simulink model "pca10040_demo"  (Simulink 7.3)
settings: Solver=ode3  SolverMode=SingleTasking  StartTime=0.0  StopTime=10.0  RelTol=1e-3
PreLoadFcn:
  | waijung.modelPreload; % Required for working with Waijung Blockset. Do not remove.
undefined symbols (not defined in the file): Blocking, In1, In2, Non, nRF52832QFAA, Out1, Out2, S132, v6
libraries: nrf5_ble_lib x4, waijung_string_manipulate x4, simulink x3, nrf5_io_lib x2, nrf5_device_config_lib x1
CloseFcn:
  | waijung.modelClose; % Required for working with Waijung Blockset. Do not remove.
settings Model: Creator=Krisada  LastModifiedBy=Navy
settings OptimizationCC: OptimizeModelRefInitCode=on  LifeSpan=1
settings HardwareCC: ProdEndianess=LittleEndian  ProdHWDeviceType=ARM Compatible->Cortex - M0  TargetEndianess=LittleEndian  TargetHWDeviceType=ARM Compatible->Cortex - M0
settings RTWCC: SystemTargetFile=nrf5.tlc  GenerateMakefile=off  TemplateMakefile=ert_default_tmf  Description=nRF5 Target  ProcessScript=nrf5_make_rtw_hook
settings CodeAppCC: IgnoreCustomStorageClasses=off
settings STFCustomTargetCC: ModelReferenceCompliant=off  CombineOutputUpdateFcns=on  ERTCustomFileBanners=on  SupportContinuousTime=off  SupportNonInlinedSFcns=off  SystemTargetFile=nrf5.tlc
settings ERTTargetCC: MultiwordLength=2048  ModelReferenceCompliant=off  ParMdlRefBuildCompliant=off  CompOptLevelCompliant=off  ERTFirstTimeCompliant=off  ModelStepFunctionPrototypeControlCompliant=off  CPPClassGenCompliant=off  InlinedParameterPlacement=NonHierarchical  ERTSrcFileBannerTemplate=nrf5_code_template.cgt  ERTHdrFileBannerTemplate=nrf5_code_template.cgt  ERTDataSrcFileTemplate=nrf5_code_template.cgt  ERTDataHdrFileTemplate=nrf5_code_template.cgt  ERTCustomFileTemplate=nrf5_file_process.tlc

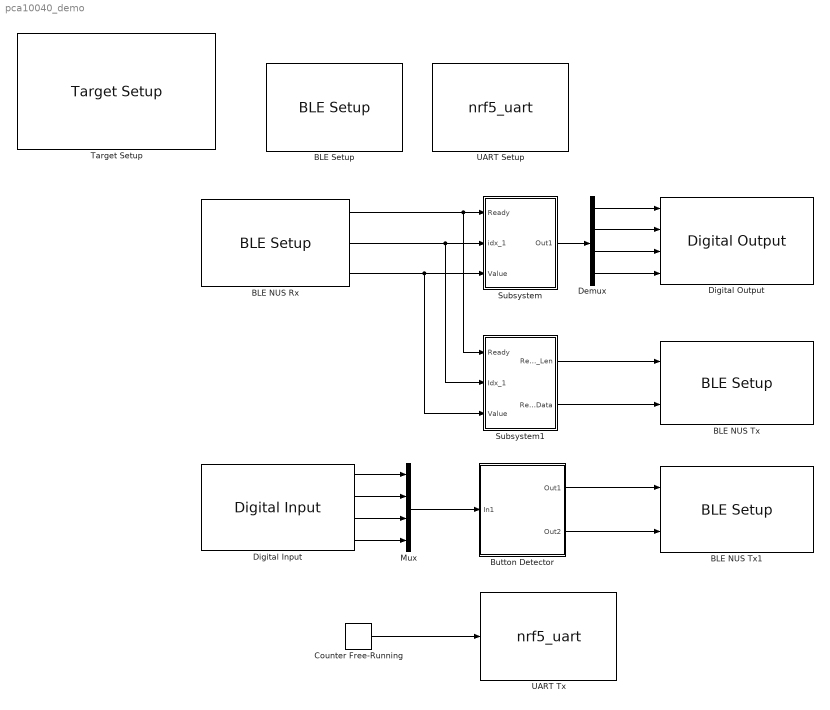
== system pca10040_demo ==
  BLE NUS Rx : nrf5_ble_lib/BLE Setup  conf=Rx  bleprofile=NUS  ble_secure_dfu=off  ble_secure_dfu_public_key='123bd49bffb387f1de3dc8dc1fc8fcce952739d331fafeb7dd16837154ace7994a0a05af319f68e2a07478477b8db746643d6dd7f5f191193738984ffcd2b963'  devicename='Nordic_UART'  advanceoptions=on  rxbuffersize=64  txbuffersize=64  transfer=Non-Blocking  packetmode=Ascii  binheader='7E 7E'  binterminator='03 03'  porttype_double=0  porttype_single=0  porttype_int8=0  porttype_uint8=3  porttype_int16=0  porttype_uint16=0  porttype_int32=0  porttype_uint32=2  asciiformat='led%d=%d'  rx_asciiterminator="CRLF (0x0D 0x0A - \"\\r\\n\")"  tx_asciiterminator=None  storagename=<empty>  portpinstr=0  sampletime=-1  enablecustomportlabel=off  cinputportlabel=In1,In2  coutputportlabel=Out1,Out2  blockid=BLENUSRx  inputporttype=[]  inputportwidth=[]  inputportlabel={}  outputporttype=[3 6 6]  outputportwidth=[]  outputportlabel={'READY' 'int32' 'int32'}  compat=0  optionstring1="[\"64\",\"64\",\"Non-Blocking\",\"Ascii\",\"led%d=%d\",\"0x0D, 0x0A\",\"2\",\"NUS\",\"Nordic_UART\",\"1\",\"0\"]"  optionstring2="[\"int32_t\",\"int32_t\"]"  optionstring3="[\"0x7E\",\"0x7E\"]"  optionstring4="[\"0x3\",\"0x3\"]"
  BLE NUS Tx : nrf5_ble_lib/BLE Setup  conf=Tx  bleprofile=NUS  ble_secure_dfu=off  ble_secure_dfu_public_key='123bd49bffb387f1de3dc8dc1fc8fcce952739d331fafeb7dd16837154ace7994a0a05af319f68e2a07478477b8db746643d6dd7f5f191193738984ffcd2b963'  devicename='Nordic_UART'  advanceoptions=on  rxbuffersize=64  txbuffersize=64  transfer=Blocking  packetmode=Raw Buffer  binheader='7E 7E'  binterminator='03 03'  porttype_double=0  porttype_single=0  porttype_int8=0  porttype_uint8=3  porttype_int16=0  porttype_uint16=0  porttype_int32=0  porttype_uint32=2  asciiformat='led%d=%d'  rx_asciiterminator="CRLF (0x0D 0x0A - \"\\r\\n\")"  tx_asciiterminator=None  storagename=<empty>  portpinstr=0  sampletime=-1  enablecustomportlabel=off  cinputportlabel=In1,In2  coutputportlabel=Out1,Out2  blockid=BLENUSTx  inputporttype=[5 3]  inputportwidth=[1 -1]  inputportlabel={'Len','Data'}  outputporttype=[]  outputportwidth=[]  outputportlabel={}  compat=0  optionstring1="[\"64\",\"64\",\"Blocking\",\"Raw Buffer\",\"led%d=%d\",\"\",\"\",\"NUS\",\"Nordic_UART\",\"1\",\"0\"]"  optionstring2="[\"int32_t\",\"int32_t\"]"  optionstring3="[\"0x7E\",\"0x7E\"]"  optionstring4="[\"0x3\",\"0x3\"]"
  BLE NUS Tx1 : nrf5_ble_lib/BLE Setup  conf=Tx  bleprofile=NUS  ble_secure_dfu=off  ble_secure_dfu_public_key='123bd49bffb387f1de3dc8dc1fc8fcce952739d331fafeb7dd16837154ace7994a0a05af319f68e2a07478477b8db746643d6dd7f5f191193738984ffcd2b963'  devicename='Nordic_UART'  advanceoptions=on  rxbuffersize=64  txbuffersize=64  transfer=Blocking  packetmode=Raw Buffer  binheader='7E 7E'  binterminator='03 03'  porttype_double=0  porttype_single=0  porttype_int8=0  porttype_uint8=3  porttype_int16=0  porttype_uint16=0  porttype_int32=0  porttype_uint32=2  asciiformat='Btn:%u,%u,%u,%u'  rx_asciiterminator="CRLF (0x0D 0x0A - \"\\r\\n\")"  tx_asciiterminator=None  storagename=<empty>  portpinstr=0  sampletime=-1  enablecustomportlabel=off  cinputportlabel=In1,In2  coutputportlabel=Out1,Out2  blockid=BLENUSTx1  inputporttype=[5 3]  inputportwidth=[1 -1]  inputportlabel={'Len','Data'}  outputporttype=[]  outputportwidth=[]  outputportlabel={}  compat=0  optionstring1="[\"64\",\"64\",\"Blocking\",\"Raw Buffer\",\"Btn:%u,%u,%u,%u\",\"\",\"\",\"NUS\",\"Nordic_UART\",\"1\",\"0\"]"  optionstring2="[\"uint32_t\",\"uint32_t\",\"uint32_t\",\"uint32_t\"]"  optionstring3="[\"0x7E\",\"0x7E\"]"  optionstring4="[\"0x3\",\"0x3\"]"
  BLE Setup : nrf5_ble_lib/BLE Setup  conf=Setup  bleprofile=NUS  ble_secure_dfu=off  ble_secure_dfu_public_key='123bd49bffb387f1de3dc8dc1fc8fcce952739d331fafeb7dd16837154ace7994a0a05af319f68e2a07478477b8db746643d6dd7f5f191193738984ffcd2b963'  devicename='aMG_BLE Demo'  advanceoptions=on  rxbuffersize=64  txbuffersize=64  transfer=Blocking  packetmode=Ascii  binheader='7E 7E'  binterminator='03 03'  porttype_double=0  porttype_single=0  porttype_int8=0  porttype_uint8=3  porttype_int16=0  porttype_uint16=0  porttype_int32=0  porttype_uint32=2  asciiformat='Value=%1.2f'  rx_asciiterminator="CRLF (0x0D 0x0A - \"\\r\\n\")"  tx_asciiterminator=None  storagename=<empty>  portpinstr=0  sampletime=-1  enablecustomportlabel=off  cinputportlabel=In1,In2  coutputportlabel=Out1,Out2  blockid=BLESetup  inputporttype=[]  inputportwidth=[]  inputportlabel={}  outputporttype=[]  outputportwidth=[]  outputportlabel={}  compat=0  optionstring1="[\"64\",\"64\",\"Blocking\",\"Ascii\",\"Value=%1.2f\",\"\",\"\",\"NUS\",\"aMG_BLE Demo\",\"1\",\"0\"]"  optionstring2="[\"float\"]"  optionstring3="[\"0x7E\",\"0x7E\"]"  optionstring4="[\"0x3\",\"0x3\"]"
  Button Detector : Subsystem
  Counter Free-Running : simulink/Sources/Counter Free-Running  SystemSampleTime=-1  NumBits=32  tsamp=-1
  Demux : Demux
  Digital Input : nrf5_io_lib/Digital Input  conf=input  port=0  drivemode=High  outputpintype=Open Drain  inputpintype=Pull Up  usepin0=off  usepin1=off  usepin2=off  usepin3=off  usepin4=off  usepin5=off  usepin6=off  usepin7=off  usepin8=off  usepin9=off  usepin10=off  usepin11=off  usepin12=off  usepin13=on  usepin14=on  usepin15=on  usepin16=on  usepin17=off  usepin18=off  usepin19=off  usepin20=off  usepin21=off  usepin22=off  usepin23=off  usepin24=off  usepin25=off  usepin26=off  usepin27=off  usepin28=off  usepin29=off  usepin30=off  usepin31=off  outputmode=uint8  sampletime=-1  enablecustomportlabel=off  cinputportlabel=In1,In2  coutputportlabel=Out1,Out2  portpinstr=off  blockid=DigitalInput  inputporttype=[]  inputportwidth=[]  inputportlabel={}  outputporttype=[3,3,3,3]  outputportwidth=[]  outputportlabel={'P0.13','P0.14','P0.15','P0.16'}  compat=0  optionstring="[\"0\",\"High\",\"PULLUP\",\"H0D1\",\"dummy\",\"dummy\",\"dummy\",\"dummy\",\"dummy\",\"dummy\",\"off\",\"off\",\"off\",\"off\",\"off\",\"off\",\"off\",\"off\",\"off\",\"off\",\"off\",\"off\",\"off\",\"on\",\"on\",\"on\",\"on\",\"off\",\"off\",\"off\",\"off\",\"off\",\"off\",\"off\",\"off\",\"off\",\"off\",\"off\",\"off\",\"off\",\"off\",\"off\"]"
  Digital Output : nrf5_io_lib/Digital Output  conf=output  port=0  drivemode=High  outputpintype=Push Pull  inputpintype=None  usepin0=off  usepin1=off  usepin2=off  usepin3=off  usepin4=off  usepin5=off  usepin6=off  usepin7=off  usepin8=off  usepin9=off  usepin10=off  usepin11=off  usepin12=off  usepin13=off  usepin14=off  usepin15=off  usepin16=off  usepin17=on  usepin18=on  usepin19=on  usepin20=on  usepin21=off  usepin22=off  usepin23=off  usepin24=off  usepin25=off  usepin26=off  usepin27=off  usepin28=off  usepin29=off  usepin30=off  usepin31=off  outputmode=uint8  sampletime=-1  enablecustomportlabel=off  cinputportlabel=In1,In2  coutputportlabel=Out1,Out2  portpinstr=off  blockid=DigitalOutput  inputporttype=[-1,-1,-1,-1]  inputportwidth=[]  inputportlabel={'P0.17','P0.18','P0.19','P0.20'}  outputporttype=[]  outputportwidth=[]  outputportlabel={}  compat=0  optionstring="[\"0\",\"High\",\"NOPULL\",\"H0H1\",\"dummy\",\"dummy\",\"dummy\",\"dummy\",\"dummy\",\"dummy\",\"off\",\"off\",\"off\",\"off\",\"off\",\"off\",\"off\",\"off\",\"off\",\"off\",\"off\",\"off\",\"off\",\"off\",\"off\",\"off\",\"off\",\"on\",\"on\",\"on\",\"on\",\"off\",\"off\",\"off\",\"off\",\"off\",\"off\",\"off\",\"off\",\"off\",\"off\",\"off\"]"
  Mux : Mux
  Subsystem : Subsystem
  Subsystem1 : Subsystem
  Target Setup : nrf5_device_config_lib/Target Setup  Priority=100  compiler=GNU ARM  previous_compiler=GNU ARM  mcu=nRF52832QFAA (S132-v6)  family=nrf52  softdevice=S132  clockconfig=None  system_nrf5_c_path=c:\users\Krisada\desktop\waijung\waijung-subversion-trunk\targets\nrf5_target\nrf5\utils\nrf5_lib\inc  lowpower=on  showmemoryconfiguration=on  stacksize=0x1000  heapsize=0x00  enableautocompiledownload=on  fullchiperase=off  ble_secure_dfu=off  ble_secure_dfu_public_key='123bd49bffb387f1de3dc8dc1fc8fcce952739d331fafeb7dd16837154ace7994a0a05af319f68e2a07478477b8db746643d6dd7f5f191193738984ffcd2b963'  programmerinterface=nrfjprog  editctrlstr=on  compilercontrolstr=-O3 -g3 -mcpu=cortex-m4 -mthumb -mabi=aapcs -Wall -mfloat-abi=hard -mfpu=fpv4-sp-d16 -ffunction-sections -fdata-sections -fno-strict-aliasing -fno-builtin -fshort-enums  assemblercontrolstr=-O3 -g3 -mcpu=cortex-m4 -mthumb -mabi=aapcs -mfloat-abi=hard -mfpu=fpv4-sp-d16  linkercontrolstr=-O3 -g3 -mthumb -mabi=aapcs -mcpu=cortex-m4 -mfloat-abi=hard -mfpu=fpv4-sp-d16 -Wl,--gc-sections --specs=nano.specs  global_define=CONFIG_GPIO_AS_PINRESET,FLOAT_ABI_HARD,NRF52,NRF52832_XXAA,NRF52_PAN_74,S132,SOFTDEVICE_PRESENT,SWI_DISABLE0,NRF_SD_BLE_API_VERSION=6  runafterdownload=on  execprofile=None  profileruart=3  profilerbaud=500000  profilertxpin=D8  profilerinitstr=0.01,168000000,1680000,500000,0  manualsetsampletime=on  sampletime=0.1  blockid=TargetSetup  systickreloadvalue=10  hseval=8000000  lastprofileruart=3  hclk=168000000  flashorigin=0x26000  flashlength=256k  ramorigin=0x200032C8  ramlength=51k  useextram=off  optionstring="[\"s132\",\"on\"]"
  UART Setup : S-Function  FunctionName=nrf5_uart  Parameters=conf,inputporttype,inputportwidth,outputporttype,outputportwidth,optionstring1,optionstring2,optionstring3,optionstring4,sampletime,blockid  EnableBusSupport=off  mask(nrf5_uart){conf=Setup, uartmodule=0, baudrate=115200, databits=8, parity=None, stopbit=1, txpin=P0.6, rxpin=P0.8, flowcontrol=None, ctspin=P0.4, rtspin=P0.2, advanceoptions=on, rxbuffersize=64, txbuffersize=64, transfer=Blocking, packetmode=Binary, binheader='7E 7E', binterminator='03 03', porttype_double=0, porttype_single=0, porttype_int8=0, porttype_uint8=0, porttype_int16=0, porttype_uint16=0, porttype_int32=0, porttype_uint32=2, asciiformat='Value=%1.2f', rx_asciiterminator=CR (0x0D - "\r"), tx_asciiterminator=CR (0x0D - "\r"), storagename=<empty>, portpinstr=0, sampletime=-1, enablecustomportlabel=off, cinputportlabel=In1,In2, coutputportlabel=Out1,Out2, blockid=UARTSetup, inputporttype=[], inputportwidth=[], inputportlabel={}, outputporttype=[], outputportwidth=[], outputportlabel={}, compat=0, optionstring1=["0","115200","6","8","None","4","2","64","64","Blocking","Binary","","0","","0","Value=%1.2f","","",""], optionstring2=["float"], optionstring3=["0x7E","0x7E"], optionstring4=["0x3","0x3"]}
      mask prompts: conf "Configuration"; uartmodule "UART Module"; baudrate "Baud rate (bps)"; databits "Data bits"; stopbit "Stop bit"; txpin "Tx Pin"; rxpin "Rx Pin"; flowcontrol "Hardware flow control"; ctspin "HW Flow control, CTS Pin"; rtspin "HW Flow control, RTS Pin"; advanceoptions "Advance options"; rxbuffersize "Rx buffer size (bytes)"; txbuffersize "Tx buffer size (bytes)"; packetmode "Packet mode"; binheader "Binary header (example: '7E 7E')"; binterminator "Binary terminator (example: '03 03')"; porttype_double "Number of data port, type DOUBLE"; porttype_single "Number of data port, type SINGLE"; porttype_int8 "Number of data port, type INT8"; porttype_uint8 "Number of data port, type UINT8"; porttype_int16 "Number of data port, type INT16"; porttype_uint16 "Number of data port, type UINT16"; porttype_int32 "Number of data port, type INT32"; porttype_uint32 "Number of data port, type UINT32"; asciiformat "Ascii format"; rx_asciiterminator "End of packet"; tx_asciiterminator "End of packet"; storagename "Buffer"; portpinstr "Port Pin String"; sampletime "Sample time (sec)"; enablecustomportlabel "Enable custom port labels"; cinputportlabel "Custom input port labels (Ex. In1, In2, In3)"; coutputportlabel "Custom output port labels (Ex. Out1, Out2, Out3)"; blockid "Block ID"; inputporttype "Input Port Type"; inputportwidth "Input Port Width"; inputportlabel "Input Port Label"; outputporttype "Output Port Type"; outputportwidth "Output Port Width"; outputportlabel "Output port label"; compat "Compatibility (Reserved for future use)"; optionstring1 "String(s) to be passed to TLC"; optionstring2 "String(s) to be passed to TLC"; optionstring3 "String(s) to be passed to TLC"; optionstring4 "String(s) to be passed to TLC"
      mask help:
      | UART Setup block.
      | Baud rate:
      |  - Valid value is 1200 to 1000000.
      mask init:
      | nrf5_uart_callback('init');
      mask Help: web(fullfile(waijungdocroot,'nrf5_uart_setup.htm'), '-browser')
      mask StyleString: popup(Setup|Tx|Rx),popup(0),edit,popup(8),popup(None|Odd|Even),popup(0.5|1|1.5|2),popup(Not used|P0.0|P0.1|P0.2|P0.3|P0.4|P0.5|P0.6|P0.7|P0.8|P0.9|P0.10|P0.11|P0.12|P0.13|P0.14|P0.15|P0.16|P0.17|P0.18|P0.19|P0.20|P0.21|P0.22|P0.23|P0.24|P0.25|P0.26|P0.27|P0.28|P0.29|P0.30|P0.31),popup(Not used|P0.0|P0.1|P0.2|P0.3|P0.4|P0.5|P0.6|P0.7|P0.8|P0.9|P0.10|P0.11|P0.12|P0.13|P0.14|P0.15|P0.16|P0.17|P0.18|P0.19|P0.20|P0.21|P0.22|P0.23|P0.24|P0.25|P0.26|P0.27|P0.28|P0.29|P0.30|P0.31),popup(None|RTS/CTS),popup(P0.0|P0.1|P0.2|P0.3|P0.4|P0.5|P0.6|P0.7|P0.8|P0.9|P0.10|P0.11|P0.12|P0.13|P0.14|P0.15|P0.16|P0.17|P0.18|P0.19|P0.20|P0.21|P0.22|P0.23|P0.24|P0.25|P0.26|P0.27|P0.28|P0.29|P0.30|P0.31),popup(P0.0|P0.1|P0.2|P0.3|P0.4|P0.5|P0.6|P0.7|P0.8|P0.9|P0.10|P0.11|P0.12|P0.13|P0.14|P0.15|P0.16|P0.17|P0.18|P0.19|P0.20|P0.21|P0.22|P0.23|P0.24|P0.25|P0.26|P0.27|P0.28|P0.29|P0.30|P0.31),checkbox,popup(16|32|64|128|256|512|1024),popup(16|32|64|128|256|512|1024),popup(Blocking|Non-Blocking),popup(Ascii|Binary|String Buffer),edit,edit,edit,edit,edit,edit,edit,edit,edit,edit,edit,popup(CR (0x0D - "\r")|LF (0x0A - "\n")|CRLF (0x0D 0x0A - "\r\n")),popup(CR (0x0D - "\r")|LF (0x0A - "\n")|CRLF (0x0D 0x0A - "\r\n")|None),popup(<empty>),edit,edit,checkbox,edit,edit,edit,edit,edit,edit,edit,edit,edit,edit,edit,edit,edit,edit
      mask CallbackString: nrf5_uart_callback('conf');||||||||nrf5_uart_callback('flowcontrol');|||nrf5_uart_callback('advanceoptions');|||nrf5_uart_callback('transfer');|nrf5_uart_callback('packetmode');|nrf5_uart_callback('binheader');|nrf5_uart_callback('binterminator');|nrf5_uart_callback('updateport');|nrf5_uart_callback('updateport');|nrf5_uart_callback('updateport');|nrf5_uart_callback('updateport');|nrf5_uart_callback('updateport');|nrf5_uart_callback('updateport');|nrf5_uart_callback('updateport');|nrf5_uart_callback('updateport');|nrf5_uart_callback('asciiformat');|||||nrf5_uart_callback('sampletime');|nrf5_uart_callback('enablecustomportlabel');|||nrf5_uart_callback('blockid');|||||||||||
      mask Display: text(0.5, 0.5, '[UART0_Setup]\nBaud: 115200\nTx/Rx buffer: 64/64\nTx/Rx pin: P0.6/P0.8','ver','middle','hor','center');
  UART Tx : S-Function  FunctionName=nrf5_uart  Parameters=conf,inputporttype,inputportwidth,outputporttype,outputportwidth,optionstring1,optionstring2,optionstring3,optionstring4,sampletime,blockid  EnableBusSupport=off  mask(nrf5_uart){conf=Tx, uartmodule=0, baudrate=115200, databits=8, parity=None, stopbit=1, txpin=P0.2, rxpin=P0.3, flowcontrol=None, ctspin=P0.4, rtspin=P0.2, advanceoptions=on, rxbuffersize=64, txbuffersize=64, transfer=Blocking, packetmode=Ascii, buffersize=32, binheader='7E 7E', binterminator='03 03', porttype_double=0, porttype_single=0, porttype_int8=0, porttype_uint8=0, porttype_int16=0, porttype_uint16=0, porttype_int32=0, porttype_uint32=2, asciiformat='Running=%u', rx_asciiterminator=CR (0x0D - "\r"), tx_asciiterminator=CRLF (0x0D 0x0A - "\r\n"), storagename=<empty>, portpinstr=0, sampletime=0.1, enablecustomportlabel=off, cinputportlabel=In1,In2, coutputportlabel=Out1,Out2, blockid=UARTTx, inputporttype=[-1], inputportwidth=[], inputportlabel={'uint32'}, outputporttype=[], outputportwidth=[], outputportlabel={}, compat=0, optionstring1=["0","115200","2","3","None","4","2","64","64","Blocking","Ascii","","0","","0","Running=%u","0x0D, 0x0A","2",""], optionstring2=["uint32_t"], optionstring3=["0x7E","0x7E"], optionstring4=["0x3","0x3"]}
      mask prompts: conf "Configuration"; uartmodule "UART Module"; baudrate "Baud rate (bps)"; databits "Data bits"; stopbit "Stop bit"; txpin "Tx Pin"; rxpin "Rx Pin"; flowcontrol "Hardware flow control"; ctspin "HW Flow control, CTS Pin"; rtspin "HW Flow control, RTS Pin"; advanceoptions "Advance options"; rxbuffersize "Rx buffer size (bytes)"; txbuffersize "Tx buffer size (bytes)"; packetmode "Packet mode"; buffersize "Buffer size"; binheader "Binary header (example: '7E 7E')"; binterminator "Binary terminator (example: '03 03')"; porttype_double "Number of data port, type DOUBLE"; porttype_single "Number of data port, type SINGLE"; porttype_int8 "Number of data port, type INT8"; porttype_uint8 "Number of data port, type UINT8"; porttype_int16 "Number of data port, type INT16"; porttype_uint16 "Number of data port, type UINT16"; porttype_int32 "Number of data port, type INT32"; porttype_uint32 "Number of data port, type UINT32"; asciiformat "Ascii format"; rx_asciiterminator "End of packet"; tx_asciiterminator "End of packet"; storagename "Buffer"; portpinstr "Port Pin String"; sampletime "Sample time (sec)"; enablecustomportlabel "Enable custom port labels"; cinputportlabel "Custom input port labels (Ex. In1, In2, In3)"; coutputportlabel "Custom output port labels (Ex. Out1, Out2, Out3)"; blockid "Block ID"; inputporttype "Input Port Type"; inputportwidth "Input Port Width"; inputportlabel "Input Port Label"; outputporttype "Output Port Type"; outputportwidth "Output Port Width"; outputportlabel "Output port label"; compat "Compatibility (Reserved for future use)"; optionstring1 "String(s) to be passed to TLC"; optionstring2 "String(s) to be passed to TLC"; optionstring3 "String(s) to be passed to TLC"; optionstring4 "String(s) to be passed to TLC"
      mask help:
      | UART Tx block.
      | For transmit data via UART communication.
      mask init:
      | nrf5_uart_callback('init');
      mask Help: web(fullfile(waijungdocroot,'nrf5_uart_tx.htm'), '-browser')
      mask StyleString: popup(Setup|Tx|Rx),popup(0),edit,popup(8),popup(None|Odd|Even),popup(0.5|1|1.5|2),popup(Not used|P0.0|P0.1|P0.2|P0.3|P0.4|P0.5|P0.6|P0.7|P0.8|P0.9|P0.10|P0.11|P0.12|P0.13|P0.14|P0.15|P0.16|P0.17|P0.18|P0.19|P0.20|P0.21|P0.22|P0.23|P0.24|P0.25|P0.26|P0.27|P0.28|P0.29|P0.30|P0.31),popup(Not used|P0.0|P0.1|P0.2|P0.3|P0.4|P0.5|P0.6|P0.7|P0.8|P0.9|P0.10|P0.11|P0.12|P0.13|P0.14|P0.15|P0.16|P0.17|P0.18|P0.19|P0.20|P0.21|P0.22|P0.23|P0.24|P0.25|P0.26|P0.27|P0.28|P0.29|P0.30|P0.31),popup(None|RTS/CTS),popup(P0.0|P0.1|P0.2|P0.3|P0.4|P0.5|P0.6|P0.7|P0.8|P0.9|P0.10|P0.11|P0.12|P0.13|P0.14|P0.15|P0.16|P0.17|P0.18|P0.19|P0.20|P0.21|P0.22|P0.23|P0.24|P0.25|P0.26|P0.27|P0.28|P0.29|P0.30|P0.31),popup(P0.0|P0.1|P0.2|P0.3|P0.4|P0.5|P0.6|P0.7|P0.8|P0.9|P0.10|P0.11|P0.12|P0.13|P0.14|P0.15|P0.16|P0.17|P0.18|P0.19|P0.20|P0.21|P0.22|P0.23|P0.24|P0.25|P0.26|P0.27|P0.28|P0.29|P0.30|P0.31),checkbox,popup(16|32|64|128|256|512|1024),popup(16|32|64|128|256|512|1024),popup(Blocking|Non-Blocking),popup(Ascii|Binary|String Buffer|Raw Buffer),popup(32|64|128|256|512|1024),edit,edit,edit,edit,edit,edit,edit,edit,edit,edit,edit,popup(CR (0x0D - "\r")|LF (0x0A - "\n")|CRLF (0x0D 0x0A - "\r\n")),popup(CR (0x0D - "\r")|LF (0x0A - "\n")|CRLF (0x0D 0x0A - "\r\n")|None),popup(<empty>),edit,edit,checkbox,edit,edit,edit,edit,edit,edit,edit,edit,edit,edit,edit,edit,edit,edit
      mask CallbackString: nrf5_uart_callback('conf');||||||||nrf5_uart_callback('flowcontrol');|||nrf5_uart_callback('advanceoptions');|||nrf5_uart_callback('transfer');|nrf5_uart_callback('packetmode');||nrf5_uart_callback('binheader');|nrf5_uart_callback('binterminator');|nrf5_uart_callback('updateport');|nrf5_uart_callback('updateport');|nrf5_uart_callback('updateport');|nrf5_uart_callback('updateport');|nrf5_uart_callback('updateport');|nrf5_uart_callback('updateport');|nrf5_uart_callback('updateport');|nrf5_uart_callback('updateport');|nrf5_uart_callback('asciiformat');|||||nrf5_uart_callback('sampletime');|nrf5_uart_callback('enablecustomportlabel');|||nrf5_uart_callback('blockid');|||||||||||
      mask Display: text(0.95, 0.5, '[UART0_Tx]\nPacket: Ascii\nTransfer: Blocking\nTs (sec): 0.1','ver','middle','hor','right'); port_label('input', 1,'uint32');
  wires:
  BLE NUS Rx/2 -> Subsystem/2(idx_1), Subsystem1/2(Idx_1)
  BLE NUS Rx/3 -> Subsystem/3(Value), Subsystem1/3(Value)
  Demux/4 -> Digital Output/4
  Demux/2 -> Digital Output/2
  Demux/3 -> Digital Output/3
  Subsystem/1(Out1) -> Demux/1
  BLE NUS Rx/1 -> Subsystem/1(Ready), Subsystem1/1(Ready)
  Subsystem1/1(Response_Len) -> BLE NUS Tx/1
  Demux/1 -> Digital Output/1
  Subsystem1/2(Response_Data) -> BLE NUS Tx/2
  Digital Input/1 -> Mux/1
  Digital Input/2 -> Mux/2
  Digital Input/3 -> Mux/3
  Digital Input/4 -> Mux/4
  Mux/1 -> Button Detector/1(In1)
  Button Detector/1(Out1) -> BLE NUS Tx1/1
  Button Detector/2(Out2) -> BLE NUS Tx1/2
  Counter Free-Running/1 -> UART Tx/1

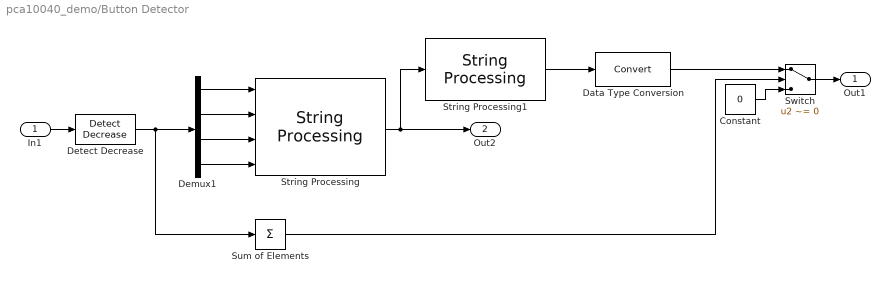
== system pca10040_demo/Button Detector ==
  In1 : Inport
  Constant : Constant  Value=0  OutDataTypeMode=uint16  OutDataType=fixdt(1, 16)  OutScaling=2^0  OutDataTypeStr=uint16  SampleTime=-1
  Data Type Conversion : DataTypeConversion  OutDataType=fixdt(1, 16)  OutScaling=2^0
  Demux1 : Demux
  Detect Decrease : simulink/Logic and Bit Operations/Detect Decrease  SystemSampleTime=-1  vinit=0.0
  String Processing : waijung_string_manipulate/String Processing  conf=processing  stringfunction=sprintf  stringformat='Btn:%u,%u,%u,%u'  begindelimiter=''  enddelimiter=''  buffersize=64  enablestatus=off  portpinstr=0  sampletime=-1  blockid=ButtonDetectorStringProcessing  inputporttype=[-1 -1 -1 -1]  inputportwidth=[1 1 1 1]  inputportlabel={'%u','%u','%u','%u'}  outputporttype=[3]  outputportwidth=[64]  outputportlabel={'Output'}  compat=0  optionstring=[]  datatypestring="[\"uint32_t\",\"uint32_t\",\"uint32_t\",\"uint32_t\"]"
  String Processing1 : waijung_string_manipulate/String Processing  conf=processing  stringfunction=strlen  stringformat='Btn:%u,%u,%u,%u'  begindelimiter=''  enddelimiter=''  buffersize=64  enablestatus=off  portpinstr=0  sampletime=-1  blockid=ButtonDetectorStringProcessing1  inputporttype=[3]  inputportwidth=[-1]  inputportlabel={'Input'}  outputporttype=[7]  outputportwidth=[1]  outputportlabel={'Length'}  compat=0  optionstring=[]  datatypestring=[]
  Sum of Elements : Sum  Inputs=+  OutDataType=fixdt(1, 16)  OutScaling=2^-10
  Switch : Switch  Criteria=u2 ~= 0  Threshold=4  OutDataType=fixdt(1, 16)  OutScaling=2^0
  Out1 : Outport
  Out2 : Outport  Port=2
  wires:
  Detect Decrease/1 -> Demux1/1, Sum of Elements/1
  Demux1/1 -> String Processing/1
  Demux1/2 -> String Processing/2
  Demux1/3 -> String Processing/3
  Demux1/4 -> String Processing/4
  String Processing/1 -> String Processing1/1, Out2/1
  Sum of Elements/1 -> Switch/2
  String Processing1/1 -> Data Type Conversion/1
  Constant/1 -> Switch/3
  Switch/1 -> Out1/1
  In1/1 -> Detect Decrease/1
  Data Type Conversion/1 -> Switch/1

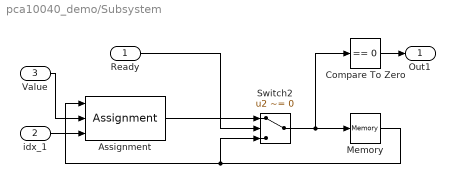
== system pca10040_demo/Subsystem ==
  Ready : Inport
  idx_1 : Inport  Port=2
  Value : Inport  Port=3
  Assignment : Assignment  IndexOptions=Index vector (port)  Indices=1  OutputSizes=1
  Compare To Zero : simulink/Logic and Bit Operations/Compare To Zero  SystemSampleTime=-1  relop===  LogicOutDataTypeMode=uint8  ZeroCross=off
  Memory : Memory  X0=[0 0 0 0]  InheritSampleTime=on  LinearizeMemory=on  LinearizeAsDelay=on
  Switch2 : Switch  Criteria=u2 ~= 0  OutDataType=fixdt(1, 16)  OutScaling=2^0
  Out1 : Outport
  wires:
  Assignment/1 -> Switch2/1
  Switch2/1 -> Memory/1, Compare To Zero/1
  Memory/1 -> Switch2/3, Assignment/1
  Value/1 -> Assignment/2
  idx_1/1 -> Assignment/3
  Compare To Zero/1 -> Out1/1
  Ready/1 -> Switch2/2

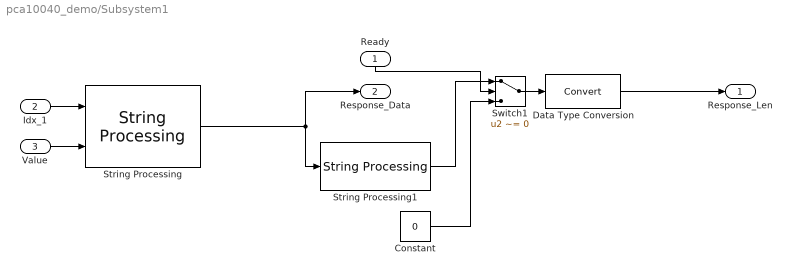
== system pca10040_demo/Subsystem1 ==
  Ready : Inport
  Idx_1 : Inport  Port=2
  Value : Inport  Port=3
  Constant : Constant  Value=0  OutDataTypeMode=uint32  OutDataType=fixdt(1, 16)  OutScaling=2^0  OutDataTypeStr=uint32  SampleTime=-1
  Data Type Conversion : DataTypeConversion  OutDataType=fixdt(1, 16)  OutScaling=2^0
  String Processing : waijung_string_manipulate/String Processing  conf=processing  stringfunction=sprintf  stringformat='OK,led%d=%d'  begindelimiter=''  enddelimiter=''  buffersize=64  enablestatus=off  portpinstr=0  sampletime=-1  blockid=Subsystem1StringProcessing  inputporttype=[-1 -1]  inputportwidth=[1 1]  inputportlabel={'%d','%d'}  outputporttype=[3]  outputportwidth=[64]  outputportlabel={'Output'}  compat=0  optionstring=[]  datatypestring="[\"int32_t\",\"int32_t\"]"
  String Processing1 : waijung_string_manipulate/String Processing  conf=processing  stringfunction=strlen  stringformat='OK,led%d=%d'  begindelimiter=''  enddelimiter=''  buffersize=64  enablestatus=off  portpinstr=0  sampletime=-1  blockid=Subsystem1StringProcessing1  inputporttype=[3]  inputportwidth=[-1]  inputportlabel={'Input'}  outputporttype=[7]  outputportwidth=[1]  outputportlabel={'Length'}  compat=0  optionstring=[]  datatypestring=[]
  Switch1 : Switch  Criteria=u2 ~= 0  OutDataType=fixdt(1, 16)  OutScaling=2^0
  Response_Len : Outport
  Response_Data : Outport  Port=2
  wires:
  String Processing/1 -> String Processing1/1, Response_Data/1
  Switch1/1 -> Data Type Conversion/1
  String Processing1/1 -> Switch1/1
  Constant/1 -> Switch1/3
  Ready/1 -> Switch1/2
  Idx_1/1 -> String Processing/1
  Value/1 -> String Processing/2
  Data Type Conversion/1 -> Response_Len/1
